simulink model "My_LQR"  (R2017a)
settings: Solver=ode45  StartTime=0.0  StopTime=60  RelTol=1e-3  EnableMultiTasking=on
PreLoadFcn:
  | load lqrpilot
undefined symbols (not defined in the file): A, B, C, D, K_lqr
settings Model: Creator=The MathWorks, Inc.  LastModifiedBy=Nizar
settings DataIOCC: LimitDataPoints=on  SaveFormat=Array
settings OptimizationCC: BlockReduction=off  BooleanDataType=off  ExpressionDepthLimit=2147483647  LifeSpan=inf
settings DebuggingCC: AlgebraicLoopMsg=none  SaveWithParameterizedLinksMsg=none  UnderspecifiedInitializationDetection=Classic  MergeDetectMultiDrivingBlocksExec=none  SignalResolutionControl=TryResolveAllWithWarning  MultiTaskDSMMsg=warning  MultiTaskCondExecSysMsg=none  FcnCallInpInsideContextMsg=warning  StateNameClashWarn=warning  SFUnexpectedBacktrackingDiag=warning  SFNoUnconditionalDefaultTransitionDiag=warning  SFExecutionAtInitializationDiag=none
settings HardwareCC: ProdBitPerPointer=32  ProdBitPerSizeT=32  ProdBitPerPtrDiffT=32  ProdLargestAtomicFloat=None  ProdIntDivRoundTo=Undefined  ProdEndianess=Unspecified  ProdWordSize=32  ProdHWDeviceType=32-bit Generic  TargetUnknown=on
settings ModelReferenceCC: PropagateSignalLabelsOutOfModel=off
settings GRTTargetCC: TargetLangStandard=C89/C90 (ANSI)  CombineOutputUpdateFcns=off  GRTInterface=on
settings ConfigComp: CovMetricSettings=dw  CovHtmlReporting=on  CovSaveCumulativeToWorkspaceVar=on  CovSaveSingleToWorkspaceVar=on  CovExternalEMLEnable=off

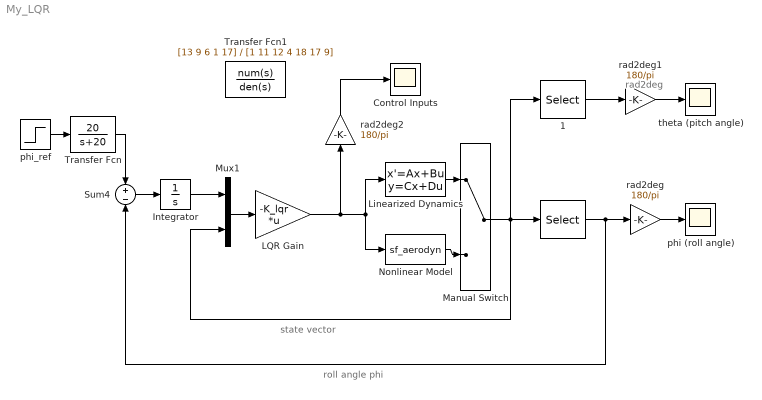
== system My_LQR ==
  note: state vector
  note: roll angle phi
  note: rad2deg
  " " : Selector  InputPortWidth=8  IndexOptions=Index vector (dialog)  Indices=8  OutputSizes=1
  " 1" : Selector  InputPortWidth=8  IndexOptions=Index vector (dialog)  Indices=7  OutputSizes=1
  Control Inputs : Scope
  Integrator : Integrator
  LQR Gain : Gain  Gain=-K_lqr  Multiplication=Matrix(K*u)  SaturateOnIntegerOverflow=on  OutDataTypeStr=Inherit: Same as input  ParamDataTypeStr=Inherit: Same as input
  Linearized Dynamics : StateSpace  A=A  B=B  C=C  D=D  X0=0
  Manual Switch : ManualSwitch
  Mux1 : Mux  Inputs=2
  Nonlinear Model : S-Function  FunctionName=sf_aerodyn  SFunctionDeploymentMode=off  EnableBusSupport=off
  Sum4 : Sum  Inputs=+-  SaturateOnIntegerOverflow=on  InputSameDT=on  OutDataTypeStr=Inherit: Same as first input
  Transfer Fcn : TransferFcn  Numerator=20  Denominator=[1 20]
  Transfer Fcn1 : TransferFcn  Numerator=[13 9 6 1 17]  Denominator=[1 11 12 4 18 17 9]
  phi (roll angle) : Scope
  phi_ref : Step  Time=0  After=pi/3  SampleTime=0
  rad2deg : Gain  Gain=180/pi  SaturateOnIntegerOverflow=on  OutDataTypeStr=Inherit: Same as input  ParamDataTypeStr=Inherit: Same as input
  rad2deg1 : Gain  Gain=180/pi  SaturateOnIntegerOverflow=on  OutDataTypeStr=Inherit: Same as input  ParamDataTypeStr=Inherit: Same as input
  rad2deg2 : Gain  Gain=180/pi  SaturateOnIntegerOverflow=on  OutDataTypeStr=Inherit: Same as input  ParamDataTypeStr=Inherit: Same as input
  theta (pitch angle) : Scope
  wires:
  phi_ref/1 -> Transfer Fcn/1
  Sum4/1 -> Integrator/1
  Mux1/1 -> LQR Gain/1
  Integrator/1 -> Mux1/1
  Transfer Fcn/1 -> Sum4/1
  LQR Gain/1 -> Linearized Dynamics/1, Nonlinear Model/1, rad2deg2/1
  Linearized Dynamics/1 -> Manual Switch/1
  Nonlinear Model/1 -> Manual Switch/2
  rad2deg/1 -> phi (roll angle)/1
  " 1"/1 -> rad2deg1/1
  rad2deg1/1 -> theta (pitch angle)/1
  rad2deg2/1 -> Control Inputs/1
  Manual Switch/1 -> " "/1, " 1"/1, Mux1/2
  " "/1 -> rad2deg/1, Sum4/2
